simulink model "Phone_A"  (R2022b)
settings: Solver=FixedStepAuto  StartTime=0.0  StopTime=10.0  RelTol=1e-3
undefined symbols (not defined in the file): _I_am_not_fine, _Longitude_limit, audio, Audio_Send, Data_Display, I_have_Fallen, Lat, Latitude_Limit_, Latitude_Send, Long, Longitude_Send, Over_accelaration, Phone_A_22b
libraries: androiduilib x9, simulink x5, androidsensorlib x3, androidaudiovideolib x3, androidcommunicationlib x3
ContinueFcn:
  | %clear m;
  | %m = mobiledev("OnePlus Nord CE 2 Lite 5G");
  | %m.MicrophoneEnabled = 0;
  | %m.MicrophoneEnabled = 1;
  | 
  | m.logging = 1;
  | pause(10);
  | m.logging = 0;
  | audTT = readAudio(m,OutputFormat="timetable");
settings Model: Creator=Zeref  LastModifiedBy=Akshat
settings OptimizationCC: EnhancedBackFolding=on  PassReuseOutputArgsAs=Individual arguments  ZeroExternalMemoryAtStartup=off  ZeroInternalMemoryAtStartup=off  MaxStackSize=64  OptimizeBlockOrder=speed  DifferentSizesBufferReuse=on  OptimizationCustomize=off  EfficientTunableParamExpr=on
settings DebuggingCC: ParameterTunabilityLossMsg=error
settings HardwareCC: ProdBitPerPointer=32  ProdBitPerSizeT=32  ProdBitPerPtrDiffT=32  ProdLargestAtomicInteger=Long  ProdLargestAtomicFloat=Double  ProdWordSize=32  ProdHWDeviceType=ARM Compatible->ARM Cortex  UseEmbeddedCoderFeatures=off
settings SFSimCC: MATLABDynamicMemAlloc=off
settings RTWCC: Description=Embedded Coder  SystemTargetFile=ert.tlc  HardwareBoard=Android Device  TLCOptions="-aInlineSetEventsForThisBaseRateFcn=TLC_FALSE -aSuppressMultiTaskScheduler=TLC_FALSE  -aRateBasedStepFcn=0"  TemplateMakefile=ert_default_tmf  RTWVerbose=off  Toolchain=Android SDK/NDK Tools
settings CodeAppCC: ForceParamTrailComments=on  IgnoreCustomStorageClasses=off  OperatorAnnotations=on  SimulinkDataObjDesc=on  SFDataObjDesc=on  InsertBlockDesc=on
settings ERTTargetCC: SupportNonInlinedSFcns=on

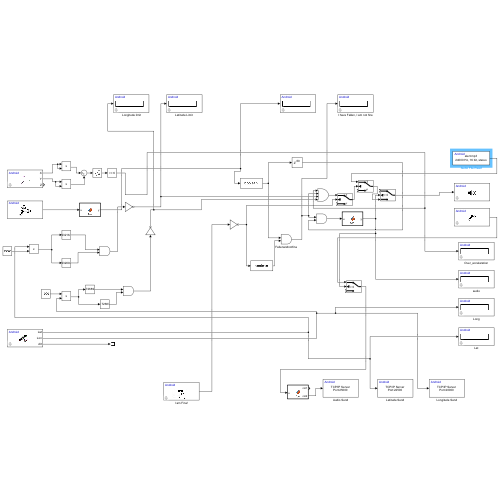
[thumbnail: Simulink's stored preview of the top-level diagram]
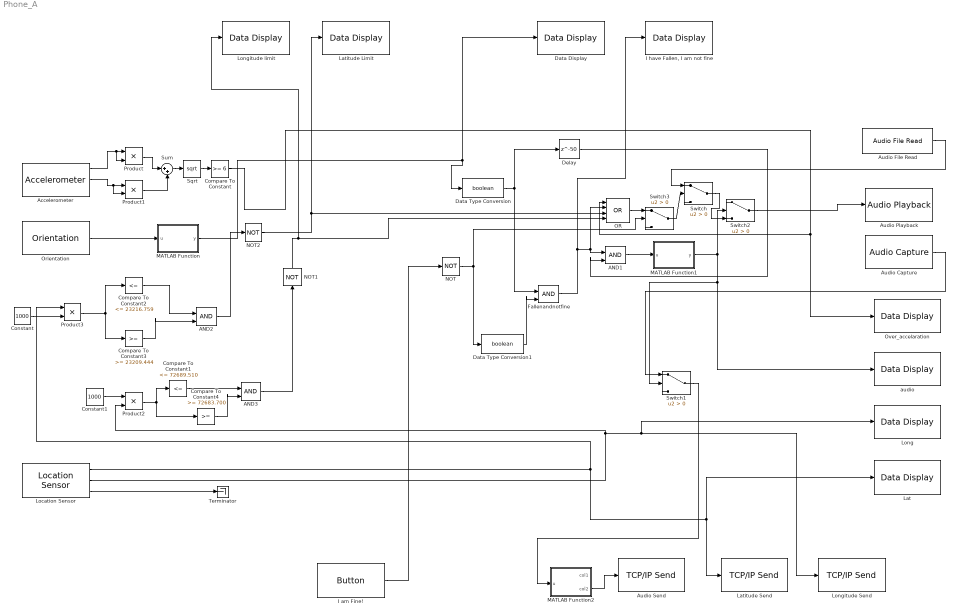
== system Phone_A ==
  " Longitude limit" : androiduilib/Data Display  DataDisplayId=Phone_A_22b/_Longitude_limit  Format=Float  Precision=6  SimulateUsing=Code generation  blockPlatform=Android
  AND1 : Logic  IconShape=distinctive  AllPortsSameDT=off  OutDataTypeStr=boolean
  AND2 : Logic  IconShape=distinctive  AllPortsSameDT=off  OutDataTypeStr=boolean
  AND3 : Logic  IconShape=distinctive  AllPortsSameDT=off  OutDataTypeStr=boolean
  Accelerometer : androidsensorlib/Accelerometer  OutputVector=off  SampleTime=0.1  BlockPlatform=Android
  Audio Capture : androidaudiovideolib/Audio Capture  SampleFreq=24000  FrameSize=30  SampleTime=0.00125  SimulateUsing=Code generation  DeviceStr=0  QueueDuration=0  BlockPlatform=Android  AudioSamplingFreq=44100
  Audio File Read : androidaudiovideolib/Audio File Read  FileName=D:\Downloads\alert.mp3  FrameSize=30
  Audio Playback : androidaudiovideolib/Audio Playback  SampleFreq=24000  AudioSamplingFreq=24000  SampleTime=0.1  DeviceStr=0  QueueDuration=0  BlockPlatform=Android
  Audio Send : androidcommunicationlib/TCP//IP Send  TCPSendId=Phone_A_22b/Audio_Send  Mode_=Server  LocalServerPort_=25000  RemoteAddr_=127.0.0.1  RemoteServerPort_=25000  ClientPortBindingSelection_=off  ClientPortToBind_=35000  BlockingMode_=off  BlockTimeout_=0.1
  Compare To Constant : simulink/Logic and Bit Operations/Compare To Constant  relop=>=  const=6  OutDataTypeStr=boolean
  Compare To Constant1 : simulink/Logic and Bit Operations/Compare To Constant  relop=<=  const=72689.510  OutDataTypeStr=boolean
  Compare To Constant2 : simulink/Logic and Bit Operations/Compare To Constant  relop=<=  const=23216.759  OutDataTypeStr=boolean
  Compare To Constant3 : simulink/Logic and Bit Operations/Compare To Constant  relop=>=  const=23209.444  OutDataTypeStr=boolean
  Compare To Constant4 : simulink/Logic and Bit Operations/Compare To Constant  relop=>=  const=72683.700  OutDataTypeStr=boolean
  Constant : Constant  Value=1000
  Constant1 : Constant  Value=1000
  Data Display : androiduilib/Data Display  DataDisplayId=Phone_A_22b/Data_Display  Format=Float  Precision=6  SimulateUsing=Code generation  blockPlatform=Android
  Data Type Conversion : DataTypeConversion  OutDataTypeStr=boolean  SaturateOnIntegerOverflow=off  RndMeth=Floor
  Data Type Conversion1 : DataTypeConversion  OutDataTypeStr=boolean  SaturateOnIntegerOverflow=off  RndMeth=Floor
  Delay : Delay  DelayLength=50  InitialCondition=0
  Fallenandnotfine : Logic  IconShape=distinctive  AllPortsSameDT=off  OutDataTypeStr=boolean
  I am Fine! : androiduilib/Button  ButtonState=Not pressed  ButtonId=Phone_A_22b/I_am_Fine!  State=off  SampleTime=0.1  BlockPlatform=Android
  "I have Fallen, I am not fine" : androiduilib/Data Display  DataDisplayId=Phone_A_22b/I_have_Fallen,_I_am_not_fine  Format=Float  Precision=6  SimulateUsing=Code generation  blockPlatform=Android
  Lat : androiduilib/Data Display  DataDisplayId=Phone_A_22b/Lat  Format=Float  Precision=6  SimulateUsing=Code generation  blockPlatform=Android
  "Latitude Limit " : androiduilib/Data Display  DataDisplayId=Phone_A_22b/Latitude_Limit_  Format=Float  Precision=6  SimulateUsing=Code generation  blockPlatform=Android
  Latitude Send : androidcommunicationlib/TCP//IP Send  TCPSendId=Phone_A_22b/Latitude_Send  Mode_=Server  LocalServerPort_=22500  RemoteAddr_=127.0.0.1  RemoteServerPort_=25000  ClientPortBindingSelection_=off  ClientPortToBind_=35000  BlockingMode_=off  BlockTimeout_=0.1
  Location Sensor : androidsensorlib/Location Sensor  OutputVector=off  SampleTime=2  BlockPlatform=Android
  Long : androiduilib/Data Display  DataDisplayId=Phone_A_22b/Long  Format=Float  Precision=6  SimulateUsing=Code generation  blockPlatform=Android
  Longitude Send : androidcommunicationlib/TCP//IP Send  TCPSendId=Phone_A_22b/Longitude_Send  Mode_=Server  LocalServerPort_=20000  RemoteAddr_=127.0.0.1  RemoteServerPort_=25000  ClientPortBindingSelection_=off  ClientPortToBind_=35000  BlockingMode_=off  BlockTimeout_=0.1
  MATLAB Function : MATLAB Function  TreatAsAtomicUnit=on
  MATLAB Function1 : MATLAB Function  TreatAsAtomicUnit=on
  MATLAB Function2 : MATLAB Function  TreatAsAtomicUnit=on
  NOT : Logic  Operator=NOT  IconShape=distinctive  AllPortsSameDT=off  OutDataTypeStr=boolean
  NOT1 : Logic  Operator=NOT  IconShape=distinctive  AllPortsSameDT=off  OutDataTypeStr=boolean
  NOT2 : Logic  Operator=NOT  IconShape=distinctive  AllPortsSameDT=off  OutDataTypeStr=boolean
  OR : Logic  Operator=OR  Inputs=4  IconShape=distinctive  AllPortsSameDT=off  OutDataTypeStr=boolean
  Orientation : androidsensorlib/Orientation  SampleTime=0.1
  Over_accelaration : androiduilib/Data Display  DataDisplayId=Phone_A_22b/Over_accelaration  Format=Float  Precision=6  SimulateUsing=Code generation  blockPlatform=Android
  Product{,1..3} (4 alike) : Product
  Sqrt : Sqrt
  Sum : Sum  Inputs=|++
  Switch{,1..3} (4 alike) : Switch  Criteria=u2 > Threshold  SaturateOnIntegerOverflow=off  InputSameDT=off
  Terminator : Terminator
  audio : androiduilib/Data Display  DataDisplayId=Phone_A_22b/audio  Format=Float  Precision=6  SimulateUsing=Code generation  blockPlatform=Android
  wires:
  AND1/1 -> MATLAB Function1/1(u)
  Data Type Conversion1/1 -> Fallenandnotfine/2
  Orientation/1 -> MATLAB Function/1(u)
  MATLAB Function1/1(y) -> Switch2/2, Switch1/2, audio/1
  Data Type Conversion/1 -> Delay/1, Fallenandnotfine/1
  Fallenandnotfine/1 -> "I have Fallen, I am not fine"/1, AND1/1, OR/2
  I am Fine!/1 -> NOT/1
  Delay/1 -> AND1/2
  NOT/1 -> Switch3/2, Data Type Conversion1/1
  Audio File Read/1 -> Switch/1
  MATLAB Function/1(y) -> Data Display/1, Data Type Conversion/1
  Audio Capture/1 -> Switch1/1
  Switch1/1 -> MATLAB Function2/1(u)
  MATLAB Function2/2(col2) -> Audio Send/1
  Switch/1 -> Switch2/3
  Location Sensor/1 -> Product3/1, Latitude Send/1, Lat/1
  Location Sensor/2 -> Product2/2, Longitude Send/1, Long/1
  Location Sensor/3 -> Terminator/1
  Accelerometer/1 -> Product/2, Product/1
  Accelerometer/2 -> Product1/2, Product1/1
  Product/1 -> Sum/1
  Product1/1 -> Sum/2
  Sum/1 -> Sqrt/1
  Sqrt/1 -> Compare To Constant/1
  Compare To Constant/1 -> Over_accelaration/1, OR/1
  Switch2/1 -> Audio Playback/1
  NOT2/1 -> "Latitude Limit "/1, OR/3
  NOT1/1 -> OR/4, " Longitude limit"/1
  Constant1/1 -> Product2/1
  Constant/1 -> Product3/2
  Product3/1 -> Compare To Constant3/1, Compare To Constant2/1
  Product2/1 -> Compare To Constant1/1, Compare To Constant4/1
  Compare To Constant2/1 -> AND2/1
  Compare To Constant3/1 -> AND2/2
  AND2/1 -> NOT2/1
  Compare To Constant1/1 -> AND3/1
  Compare To Constant4/1 -> AND3/2
  AND3/1 -> NOT1/1
  OR/1 -> Switch3/1
  Switch3/1 -> Switch/2

== matlab function Phone_A/MATLAB Function ==
  data: u input; y output
function y = fcn(u)

k = u(2);
if k<-60 || k>60
    y = 1;
else
    y = 0;
end

== matlab function Phone_A/MATLAB Function2 ==
  data: u input; col1 output; col2 output
function [col1,col2] = fcn(u)
    col1 = u(:,1);
    col2 = u(:,2);
end

== matlab function Phone_A/MATLAB Function1 ==
  data: u input; y output
function y = fcn(u)
    if u == true
        y = 1;
    else
        y = 0;
    end
